simulink model "Three-phase Asynchronous Motor_Speed Regulation"  (R2017b)
settings: Solver=ode23tb  StartTime=0.0  StopTime=9  MaxStep=1e-4  RelTol=1e-3
libraries: powerlib x51, powerlib_meascontrol x1, simulink x1
settings Model: Creator=13248  LastModifiedBy=13248
settings DebuggingCC: UnconnectedInputMsg=none  UnconnectedOutputMsg=none  UnconnectedLineMsg=none

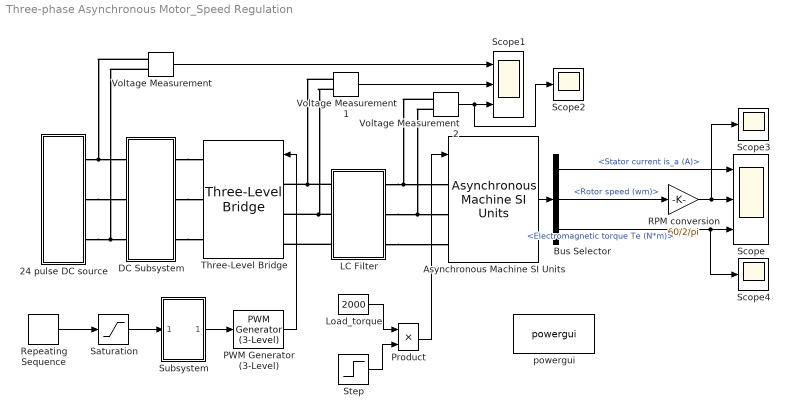
== system Three-phase Asynchronous Motor_Speed Regulation ==
  " DC Subsystem" : Subsystem
  24 pulse DC source : Subsystem
  Asynchronous Machine SI Units : powerlib/Machines/Asynchronous Machine SI Units  RotorType=Squirrel-cage  PresetModel=No  MechanicalLoad=Torque Tm  ShowDetailedParameters=on  ReferenceFrame=Rotor  Units=SI  MeasurementBus=off  NominalParameters=[500e3 6000 50]  Stator=[2 7/314]  Rotor=[1.9 5/314]  Cage1=[0.4155 0.002066]  Cage2=[0.4168 0.0003495]  Lm=235/314  Mechanical=[48 0 2]  PolePairs=2  InitialConditions=[1,0 0,0,0 0,0,0]  SimulateSaturation=off  Saturation=[14.03593122, 27.81365428, 53.79336849, 72.68890987, 97.98006896, 148.6815601, 215.7428561, 302.9841135, 428.7778367 ; 230, 322, 414, 460, 506, 552, 598, 644, 690]  LoadFlowParameters=1492000  TsPowergui=0  TsBlock=-1  IterativeModel=Trapezoidal non iterative  IterativeDiscreteModel=Trapezoidal non iterative  Pmec=1.492e+006
  Bus Selector : BusSelector  OutputSignals=Stator measurements.Stator current is_a (A),Mechanical.Rotor speed (wm),Mechanical.Electromagnetic torque Te (N*m)
  LC Filter : Subsystem
  Load_torque : Constant  Value=2000
  PWM Generator (3-Level) : powerlib_meascontrol/Pulse & Signal Generators/PWM Generator (3-Level)  ModulatorType=Three-phase bridge (12 pulses)  ModulatorMode=Unsynchronized  nF=27  Fc=18*50  ModulatingSignals=off  m=0.8  Freq=60  Phase=0  Ts=0
      settings: SourceProductName=Simscape Power Systems  SourceProductBaseCode=PS
  Product : Product
  RPM conversion : Gain  Gain=60/2/pi
  Repeating Sequence : simulink/Sources/Repeating Sequence  rep_seq_t=[0,0.5,2.5,2.51,5,5.01,10]  rep_seq_y=[0 15 15 35 35 50 50]
  Saturation : Saturate  UpperLimit=60  LowerLimit=0
  Scope : Scope  NumInputPorts=3
  Scope1 : Scope  NumInputPorts=3
  Scope2 : Scope
  Scope3 : Scope
  Scope4 : Scope
  Step : Step  Time=1.5  SampleTime=0
  Subsystem : Subsystem
  Three-Level Bridge : powerlib/Power Electronics/Three-Level Bridge  Arms=3  SnubberResistance=1e6  SbubberCapacitance=inf  Device=GTO / Diodes  Ron=1e-4  ForwardVoltages="[  1  1  ]"  Measurements=None
      settings: SourceProductName=Simscape Power Systems  SourceProductBaseCode=PS
  Voltage Measurement : powerlib/Measurements/Voltage Measurement  PhasorSimulation=off  OutputType=Complex  PSBequivalent=0
  Voltage Measurement1 : powerlib/Measurements/Voltage Measurement  PhasorSimulation=off  OutputType=Complex  PSBequivalent=0
  Voltage Measurement2 : powerlib/Measurements/Voltage Measurement  PhasorSimulation=off  OutputType=Complex  PSBequivalent=0
  powergui : powerlib/powergui  Priority=1  SimulationMode=Discrete  SampleTime=5.144e-6  frequency=60  Iterations=50  frequencyindice=50  Pbase=100e6  ErrMax=1e-4  UnitsV=kV  UnitsW=MW  buscounter=0  FunctionMessages=off  echomessages=off  EnableUseOfTLC=off  CurrentSourceSwitches=off  DisableSnubberDevices=off  DisableRonSwitches=off  DisableVfSwitches=off  DisplayEquations=off  SolverType=Tustin/Backward Euler (TBE)  Interpol=off  ExternalGateDelay=off  methode=off  Ts=100  x0status=steady  SPID=on  SwTol=0  HookPort=off  RestoreLinks=warning  ResistiveCurrentMeasurement=off  Frange=[0:2:500]  Ylog=off  Xlog=on  ShowGrid=off  save=off  variable=ZData  structure=0  ZoomFFT=off  StartTime=0.0  cycles=1  DisplayStyle=1  fundamental=60  FreqAxis=off  MaxFrequency=1000  frequencyindicesteady=1  RmsSteady=1  display=off
  wires:
  Bus Selector/2 -> RPM conversion/1  "<Rotor speed (wm)>"
  RPM conversion/1 -> Scope3/1, Scope/2
  Bus Selector/3 -> Scope/3, Scope4/1  "<Electromagnetic torque Te (N*m)>"
  Bus Selector/1 -> Scope/1  "<Stator current is_a (A)>"
  Repeating Sequence/1 -> Saturation/1
  Saturation/1 -> Subsystem/1(Cmd)
  Subsystem/1(Ust) -> PWM Generator (3-Level)/1
  PWM Generator (3-Level)/1 -> Three-Level Bridge/1
  Asynchronous Machine SI Units/1 -> Bus Selector/1
  Product/1 -> Asynchronous Machine SI Units/1
  Load_torque/1 -> Product/1
  Step/1 -> Product/2
  Voltage Measurement/1 -> Scope1/1
  Voltage Measurement1/1 -> Scope1/2
  Voltage Measurement2/1 -> Scope2/1, Scope1/3
  connections:
  24 pulse DC source/RConn1 -- Voltage Measurement/LConn1 -- " DC Subsystem"/LConn1
  24 pulse DC source/RConn2 -- " DC Subsystem"/LConn2
  24 pulse DC source/RConn3 -- Voltage Measurement/LConn2 -- " DC Subsystem"/LConn3
  " DC Subsystem"/RConn1 -- Three-Level Bridge/RConn1
  " DC Subsystem"/RConn2 -- Three-Level Bridge/RConn2
  " DC Subsystem"/RConn3 -- Three-Level Bridge/RConn3
  LC Filter/LConn1 -- Three-Level Bridge/LConn1 -- Voltage Measurement1/LConn1
  LC Filter/LConn2 -- Three-Level Bridge/LConn2 -- Voltage Measurement1/LConn2
  LC Filter/LConn3 -- Three-Level Bridge/LConn3
  LC Filter/RConn1 -- Voltage Measurement2/LConn1 -- Asynchronous Machine SI Units/LConn1
  LC Filter/RConn2 -- Voltage Measurement2/LConn2 -- Asynchronous Machine SI Units/LConn2
  LC Filter/RConn3 -- Asynchronous Machine SI Units/LConn3

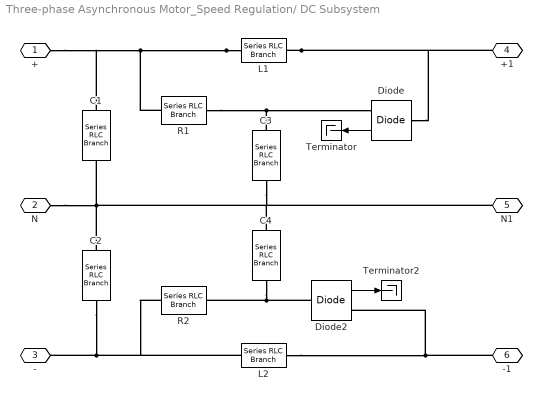
== system Three-phase Asynchronous Motor_Speed Regulation/ DC Subsystem ==
  C1 : powerlib/Elements/Series RLC Branch  LConnTagsString=__new0  RConnTagsString=__new0  BranchType=C  Resistance=0.5  Inductance=15e-6  SetiL0=off  InitialCurrent=0  Capacitance=960e-6  Setx0=off  InitialVoltage=0  Measurements=None
  C2 : powerlib/Elements/Series RLC Branch  LConnTagsString=__new0  RConnTagsString=__new0  BranchType=C  Resistance=0.5  Inductance=15e-6  SetiL0=off  InitialCurrent=0  Capacitance=960e-6  Setx0=off  InitialVoltage=0  Measurements=None
  C3 : powerlib/Elements/Series RLC Branch  LConnTagsString=__new0  RConnTagsString=__new0  BranchType=C  Resistance=0.5  Inductance=15e-6  SetiL0=off  InitialCurrent=0  Capacitance=10e-6  Setx0=off  InitialVoltage=0  Measurements=None
  C4 : powerlib/Elements/Series RLC Branch  LConnTagsString=__new0  RConnTagsString=__new0  BranchType=C  Resistance=0.5  Inductance=15e-6  SetiL0=off  InitialCurrent=0  Capacitance=10e-6  Setx0=off  InitialVoltage=0  Measurements=None
  Diode : powerlib/Power Electronics/Diode  Ron=0.001  Lon=0  Vf=0.8  IC=0  UseSnubber=0  Rs=500  Cs=250e-9  Measurements=on
  Diode2 : powerlib/Power Electronics/Diode  Ron=0.001  Lon=0  Vf=0.8  IC=0  UseSnubber=0  Rs=500  Cs=250e-9  Measurements=on
  L1 : powerlib/Elements/Series RLC Branch  LConnTagsString=__new0  RConnTagsString=__new0  BranchType=L  Resistance=1  Inductance=15e-6  SetiL0=off  InitialCurrent=0  Capacitance=1e-6  Setx0=off  InitialVoltage=0  Measurements=None
  L2 : powerlib/Elements/Series RLC Branch  LConnTagsString=__new0  RConnTagsString=__new0  BranchType=L  Resistance=1  Inductance=15e-6  SetiL0=off  InitialCurrent=0  Capacitance=1e-6  Setx0=off  InitialVoltage=0  Measurements=None
  R1 : powerlib/Elements/Series RLC Branch  LConnTagsString=__new0  RConnTagsString=__new0  BranchType=R  Resistance=0.5  Inductance=15e-6  SetiL0=off  InitialCurrent=0  Capacitance=1e-6  Setx0=off  InitialVoltage=0  Measurements=None
  R2 : powerlib/Elements/Series RLC Branch  LConnTagsString=__new0  RConnTagsString=__new0  BranchType=R  Resistance=0.5  Inductance=15e-6  SetiL0=off  InitialCurrent=0  Capacitance=1e-6  Setx0=off  InitialVoltage=0  Measurements=None
  Terminator : Terminator
  Terminator2 : Terminator
  + : PMIOPort  Port=1  Side=Left
  N : PMIOPort  Port=2  Side=Left
  - : PMIOPort  Port=3  Side=Left
  +1 : PMIOPort  Port=4  Side=Right
  N1 : PMIOPort  Port=5  Side=Right
  -1 : PMIOPort  Port=6  Side=Right
  wires:
  Diode2/1 -> Terminator2/1
  Diode/1 -> Terminator/1
  connections:
  L1/RConn1 -- +1/RConn1 -- Diode/LConn1
  R1/RConn1 -- C3/LConn1 -- Diode/RConn1
  L1/LConn1 -- +/RConn1 -- C1/LConn1 -- R1/LConn1
  C2/RConn1 -- -/RConn1 -- R2/LConn1 -- L2/LConn1
  C4/RConn1 -- Diode2/LConn1 -- R2/RConn1
  C2/LConn1 -- N/RConn1 -- N1/RConn1 -- C4/LConn1 -- C3/RConn1 -- C1/RConn1
  L2/RConn1 -- -1/RConn1 -- Diode2/RConn1

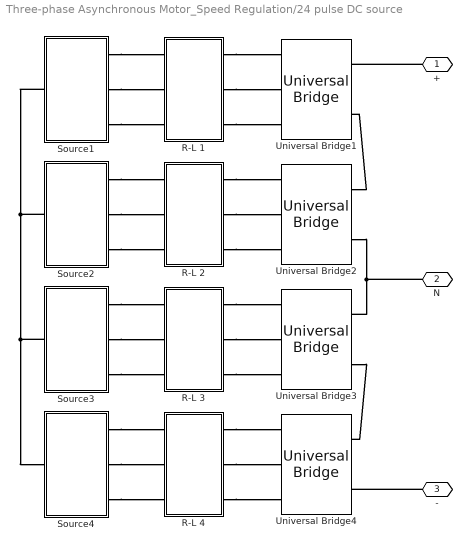
== system Three-phase Asynchronous Motor_Speed Regulation/24 pulse DC source ==
  R-L 1 : Subsystem
  R-L 2 : Subsystem
  R-L 3 : Subsystem
  R-L 4 : Subsystem
  Source1 : Subsystem
  Source2 : Subsystem
  Source3 : Subsystem
  Source4 : Subsystem
  Universal Bridge{1..4} (4 alike) : powerlib/Power Electronics/Universal Bridge  Arms=3  SnubberResistance=250  SnubberCapacitance=0.1e-6  Device=Diodes  Ron=0.01  Lon=0  ForwardVoltages="[  0  0  ]"  ForwardVoltage=0.8  GTOparameters=[ 10e-6 , 20e-6 ]  IGBTparameters=[ 1e-6 , 2e-6 ]  Measurements=Device currents  Measurements_2=None  converterType=Rectifier
  + : PMIOPort  Port=1  Side=Right
  N : PMIOPort  Port=2  Side=Right
  - : PMIOPort  Port=3  Side=Right
  connections:
  Source1/RConn2 -- R-L 1/LConn2
  R-L 2/RConn3 -- Universal Bridge2/LConn3
  R-L 2/RConn1 -- Universal Bridge2/LConn1
  Source1/LConn1 -- Source2/LConn1 -- Source3/LConn1 -- Source4/LConn1
  Universal Bridge3/RConn2 -- Universal Bridge4/RConn1
  Source1/RConn3 -- R-L 1/LConn3
  R-L 1/RConn3 -- Universal Bridge1/LConn3
  R-L 1/RConn2 -- Universal Bridge1/LConn2
  R-L 2/RConn2 -- Universal Bridge2/LConn2
  -/RConn1 -- Universal Bridge4/RConn2
  R-L 3/RConn1 -- Universal Bridge3/LConn1
  R-L 3/RConn2 -- Universal Bridge3/LConn2
  R-L 4/RConn1 -- Universal Bridge4/LConn1
  R-L 4/RConn2 -- Universal Bridge4/LConn2
  Universal Bridge2/RConn2 -- N/RConn1 -- Universal Bridge3/RConn1
  R-L 4/RConn3 -- Universal Bridge4/LConn3
  Source2/RConn2 -- R-L 2/LConn2
  Source4/RConn3 -- R-L 4/LConn3
  Source2/RConn1 -- R-L 2/LConn1
  R-L 1/RConn1 -- Universal Bridge1/LConn1
  Source4/RConn2 -- R-L 4/LConn2
  Source1/RConn1 -- R-L 1/LConn1
  R-L 3/RConn3 -- Universal Bridge3/LConn3
  +/RConn1 -- Universal Bridge1/RConn1
  Universal Bridge2/RConn1 -- Universal Bridge1/RConn2
  Source3/RConn3 -- R-L 3/LConn3
  Source4/RConn1 -- R-L 4/LConn1
  Source3/RConn2 -- R-L 3/LConn2
  Source3/RConn1 -- R-L 3/LConn1
  Source2/RConn3 -- R-L 2/LConn3

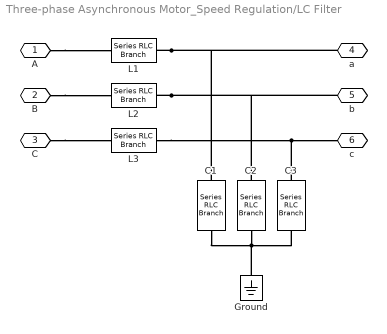
== system Three-phase Asynchronous Motor_Speed Regulation/LC Filter ==
  C1 : powerlib/Elements/Series RLC Branch  LConnTagsString=__new0  RConnTagsString=__new0  BranchType=C  Resistance=0.5  Inductance=15e-6  SetiL0=off  InitialCurrent=0  Capacitance=120e-6  Setx0=off  InitialVoltage=0  Measurements=None
  C2 : powerlib/Elements/Series RLC Branch  LConnTagsString=__new0  RConnTagsString=__new0  BranchType=C  Resistance=0.5  Inductance=15e-6  SetiL0=off  InitialCurrent=0  Capacitance=120e-6  Setx0=off  InitialVoltage=0  Measurements=None
  C3 : powerlib/Elements/Series RLC Branch  LConnTagsString=__new0  RConnTagsString=__new0  BranchType=C  Resistance=0.5  Inductance=15e-6  SetiL0=off  InitialCurrent=0  Capacitance=120e-6  Setx0=off  InitialVoltage=0  Measurements=None
  Ground : powerlib/Elements/Ground  LConnTagsString=a
  L1 : powerlib/Elements/Series RLC Branch  LConnTagsString=__new0  RConnTagsString=__new0  BranchType=L  Resistance=1  Inductance=0.002  SetiL0=off  InitialCurrent=0  Capacitance=1e-6  Setx0=off  InitialVoltage=0  Measurements=None
  L2 : powerlib/Elements/Series RLC Branch  LConnTagsString=__new0  RConnTagsString=__new0  BranchType=L  Resistance=1  Inductance=0.002  SetiL0=off  InitialCurrent=0  Capacitance=1e-6  Setx0=off  InitialVoltage=0  Measurements=None
  L3 : powerlib/Elements/Series RLC Branch  LConnTagsString=__new0  RConnTagsString=__new0  BranchType=L  Resistance=1  Inductance=0.002  SetiL0=off  InitialCurrent=0  Capacitance=1e-6  Setx0=off  InitialVoltage=0  Measurements=None
  A : PMIOPort  Port=1  Side=Left
  B : PMIOPort  Port=2  Side=Left
  C : PMIOPort  Port=3  Side=Left
  a : PMIOPort  Port=4  Side=Right
  b : PMIOPort  Port=5  Side=Right
  c : PMIOPort  Port=6  Side=Right
  connections:
  L3/RConn1 -- c/RConn1 -- C3/LConn1
  L1/RConn1 -- a/RConn1 -- C1/LConn1
  C2/RConn1 -- Ground/LConn1 -- C3/RConn1 -- C1/RConn1
  L2/RConn1 -- b/RConn1 -- C2/LConn1
  B/RConn1 -- L2/LConn1
  A/RConn1 -- L1/LConn1
  C/RConn1 -- L3/LConn1

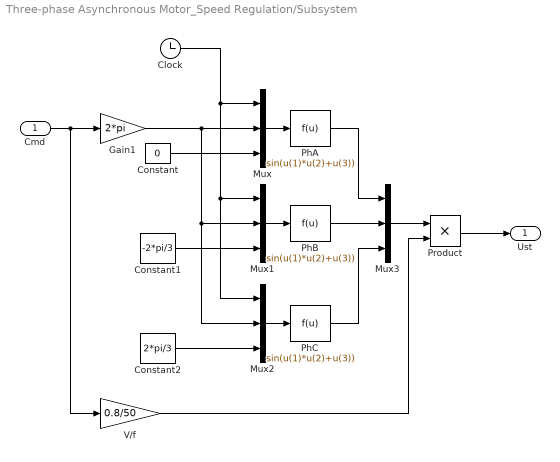
== system Three-phase Asynchronous Motor_Speed Regulation/Subsystem ==
  Cmd : Inport
  Clock : Clock
  Constant : Constant  Value=0
  Constant1 : Constant  Value=-2*pi/3
  Constant2 : Constant  Value=2*pi/3
  Gain1 : Gain  Gain=2*pi
  Mux{,1..3} (4 alike) : Mux  Inputs=3
  PhA : Fcn  Expr=sin(u(1)*u(2)+u(3))
  PhB : Fcn  Expr=sin(u(1)*u(2)+u(3))
  PhC : Fcn  Expr=sin(u(1)*u(2)+u(3))
  Product : Product
  V/f : Gain  Gain=0.8/50
  Ust : Outport
  wires:
  V/f/1 -> Product/2
  Constant2/1 -> Mux2/3
  Product/1 -> Ust/1
  Constant/1 -> Mux/3
  Clock/1 -> Mux2/1, Mux1/1, Mux/1
  PhC/1 -> Mux3/3
  Cmd/1 -> V/f/1, Gain1/1
  Mux3/1 -> Product/1
  Mux1/1 -> PhB/1
  Constant1/1 -> Mux1/3
  Mux2/1 -> PhC/1
  PhB/1 -> Mux3/2
  PhA/1 -> Mux3/1
  Mux/1 -> PhA/1
  Gain1/1 -> Mux2/2, Mux1/2, Mux/2

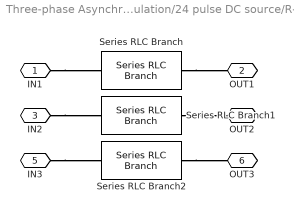
== system Three-phase Asynchronous Motor_Speed Regulation/24 pulse DC source/R-L 1 ==
  Series RLC Branch : powerlib/Elements/Series RLC Branch  LConnTagsString=__new0  RConnTagsString=__new0  BranchType=RL  Resistance=0.9  Inductance=0.002  SetiL0=off  InitialCurrent=0  Capacitance=1e-6  Setx0=off  InitialVoltage=0  Measurements=None
  Series RLC Branch1 : powerlib/Elements/Series RLC Branch  LConnTagsString=__new0  RConnTagsString=__new0  BranchType=RL  Resistance=0.9  Inductance=0.002  SetiL0=off  InitialCurrent=0  Capacitance=1e-6  Setx0=off  InitialVoltage=0  Measurements=None
  Series RLC Branch2 : powerlib/Elements/Series RLC Branch  LConnTagsString=__new0  RConnTagsString=__new0  BranchType=RL  Resistance=0.9  Inductance=0.002  SetiL0=off  InitialCurrent=0  Capacitance=1e-6  Setx0=off  InitialVoltage=0  Measurements=None
  IN1 : PMIOPort  Port=1  Side=Left
  OUT1 : PMIOPort  Port=2  Side=Right
  IN2 : PMIOPort  Port=3  Side=Left
  OUT2 : PMIOPort  Port=4  Side=Right
  IN3 : PMIOPort  Port=5  Side=Left
  OUT3 : PMIOPort  Port=6  Side=Right
  connections:
  IN2/RConn1 -- Series RLC Branch1/LConn1
  Series RLC Branch1/RConn1 -- OUT2/RConn1
  IN1/RConn1 -- Series RLC Branch/LConn1
  Series RLC Branch/RConn1 -- OUT1/RConn1
  IN3/RConn1 -- Series RLC Branch2/LConn1
  Series RLC Branch2/RConn1 -- OUT3/RConn1

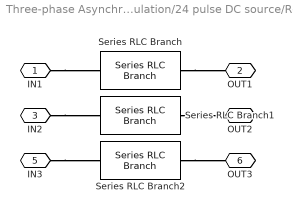
== system Three-phase Asynchronous Motor_Speed Regulation/24 pulse DC source/R-L 2 ==
  Series RLC Branch : powerlib/Elements/Series RLC Branch  LConnTagsString=__new0  RConnTagsString=__new0  BranchType=RL  Resistance=0.9  Inductance=0.002  SetiL0=off  InitialCurrent=0  Capacitance=1e-6  Setx0=off  InitialVoltage=0  Measurements=None
  Series RLC Branch1 : powerlib/Elements/Series RLC Branch  LConnTagsString=__new0  RConnTagsString=__new0  BranchType=RL  Resistance=0.9  Inductance=0.002  SetiL0=off  InitialCurrent=0  Capacitance=1e-6  Setx0=off  InitialVoltage=0  Measurements=None
  Series RLC Branch2 : powerlib/Elements/Series RLC Branch  LConnTagsString=__new0  RConnTagsString=__new0  BranchType=RL  Resistance=0.9  Inductance=0.002  SetiL0=off  InitialCurrent=0  Capacitance=1e-6  Setx0=off  InitialVoltage=0  Measurements=None
  IN1 : PMIOPort  Port=1  Side=Left
  OUT1 : PMIOPort  Port=2  Side=Right
  IN2 : PMIOPort  Port=3  Side=Left
  OUT2 : PMIOPort  Port=4  Side=Right
  IN3 : PMIOPort  Port=5  Side=Left
  OUT3 : PMIOPort  Port=6  Side=Right
  connections:
  IN2/RConn1 -- Series RLC Branch1/LConn1
  Series RLC Branch1/RConn1 -- OUT2/RConn1
  IN1/RConn1 -- Series RLC Branch/LConn1
  Series RLC Branch/RConn1 -- OUT1/RConn1
  IN3/RConn1 -- Series RLC Branch2/LConn1
  Series RLC Branch2/RConn1 -- OUT3/RConn1

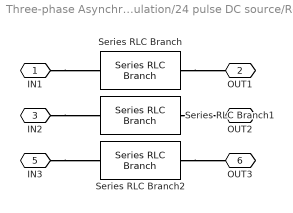
== system Three-phase Asynchronous Motor_Speed Regulation/24 pulse DC source/R-L 3 ==
  Series RLC Branch : powerlib/Elements/Series RLC Branch  LConnTagsString=__new0  RConnTagsString=__new0  BranchType=RL  Resistance=0.9  Inductance=0.002  SetiL0=off  InitialCurrent=0  Capacitance=1e-6  Setx0=off  InitialVoltage=0  Measurements=None
  Series RLC Branch1 : powerlib/Elements/Series RLC Branch  LConnTagsString=__new0  RConnTagsString=__new0  BranchType=RL  Resistance=0.9  Inductance=0.002  SetiL0=off  InitialCurrent=0  Capacitance=1e-6  Setx0=off  InitialVoltage=0  Measurements=None
  Series RLC Branch2 : powerlib/Elements/Series RLC Branch  LConnTagsString=__new0  RConnTagsString=__new0  BranchType=RL  Resistance=0.9  Inductance=0.002  SetiL0=off  InitialCurrent=0  Capacitance=1e-6  Setx0=off  InitialVoltage=0  Measurements=None
  IN1 : PMIOPort  Port=1  Side=Left
  OUT1 : PMIOPort  Port=2  Side=Right
  IN2 : PMIOPort  Port=3  Side=Left
  OUT2 : PMIOPort  Port=4  Side=Right
  IN3 : PMIOPort  Port=5  Side=Left
  OUT3 : PMIOPort  Port=6  Side=Right
  connections:
  IN2/RConn1 -- Series RLC Branch1/LConn1
  Series RLC Branch1/RConn1 -- OUT2/RConn1
  IN1/RConn1 -- Series RLC Branch/LConn1
  Series RLC Branch/RConn1 -- OUT1/RConn1
  IN3/RConn1 -- Series RLC Branch2/LConn1
  Series RLC Branch2/RConn1 -- OUT3/RConn1

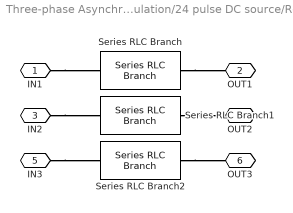
== system Three-phase Asynchronous Motor_Speed Regulation/24 pulse DC source/R-L 4 ==
  Series RLC Branch : powerlib/Elements/Series RLC Branch  LConnTagsString=__new0  RConnTagsString=__new0  BranchType=RL  Resistance=0.9  Inductance=0.002  SetiL0=off  InitialCurrent=0  Capacitance=1e-6  Setx0=off  InitialVoltage=0  Measurements=None
  Series RLC Branch1 : powerlib/Elements/Series RLC Branch  LConnTagsString=__new0  RConnTagsString=__new0  BranchType=RL  Resistance=0.9  Inductance=0.002  SetiL0=off  InitialCurrent=0  Capacitance=1e-6  Setx0=off  InitialVoltage=0  Measurements=None
  Series RLC Branch2 : powerlib/Elements/Series RLC Branch  LConnTagsString=__new0  RConnTagsString=__new0  BranchType=RL  Resistance=0.9  Inductance=0.002  SetiL0=off  InitialCurrent=0  Capacitance=1e-6  Setx0=off  InitialVoltage=0  Measurements=None
  IN1 : PMIOPort  Port=1  Side=Left
  OUT1 : PMIOPort  Port=2  Side=Right
  IN2 : PMIOPort  Port=3  Side=Left
  OUT2 : PMIOPort  Port=4  Side=Right
  IN3 : PMIOPort  Port=5  Side=Left
  OUT3 : PMIOPort  Port=6  Side=Right
  connections:
  IN2/RConn1 -- Series RLC Branch1/LConn1
  Series RLC Branch1/RConn1 -- OUT2/RConn1
  IN1/RConn1 -- Series RLC Branch/LConn1
  Series RLC Branch/RConn1 -- OUT1/RConn1
  IN3/RConn1 -- Series RLC Branch2/LConn1
  Series RLC Branch2/RConn1 -- OUT3/RConn1

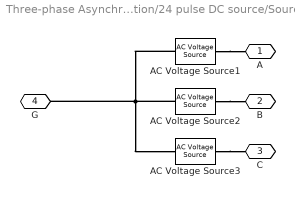
== system Three-phase Asynchronous Motor_Speed Regulation/24 pulse DC source/Source1 ==
  AC Voltage Source1 : powerlib/Electrical Sources/AC Voltage Source  Amplitude=6600/sqrt(3)*sqrt(2)  Phase=0  Frequency=50  SampleTime=0  Measurements=None  BusType=swing  Pref=10e3  Qref=0  Qmin=-inf  Qmax=+inf
  AC Voltage Source2 : powerlib/Electrical Sources/AC Voltage Source  Amplitude=6600/sqrt(3)*sqrt(2)  Phase=-120  Frequency=50  SampleTime=0  Measurements=None  BusType=swing  Pref=10e3  Qref=0  Qmin=-inf  Qmax=+inf
  AC Voltage Source3 : powerlib/Electrical Sources/AC Voltage Source  Amplitude=6600/sqrt(3)*sqrt(2)  Phase=120  Frequency=50  SampleTime=0  Measurements=None  BusType=swing  Pref=10e3  Qref=0  Qmin=-inf  Qmax=+inf
  A : PMIOPort  Port=1  Side=Right
  B : PMIOPort  Port=2  Side=Right
  C : PMIOPort  Port=3  Side=Right
  G : PMIOPort  Port=4  Side=Left
  connections:
  AC Voltage Source1/LConn1 -- G/RConn1 -- AC Voltage Source2/LConn1 -- AC Voltage Source3/LConn1
  AC Voltage Source3/RConn1 -- C/RConn1
  AC Voltage Source2/RConn1 -- B/RConn1
  AC Voltage Source1/RConn1 -- A/RConn1

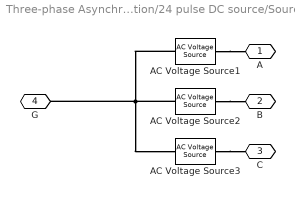
== system Three-phase Asynchronous Motor_Speed Regulation/24 pulse DC source/Source2 ==
  AC Voltage Source1 : powerlib/Electrical Sources/AC Voltage Source  Amplitude=6600/sqrt(3)*sqrt(2)  Phase=15  Frequency=50  SampleTime=0  Measurements=None  BusType=swing  Pref=10e3  Qref=0  Qmin=-inf  Qmax=+inf
  AC Voltage Source2 : powerlib/Electrical Sources/AC Voltage Source  Amplitude=6600/sqrt(3)*sqrt(2)  Phase=-105  Frequency=50  SampleTime=0  Measurements=None  BusType=swing  Pref=10e3  Qref=0  Qmin=-inf  Qmax=+inf
  AC Voltage Source3 : powerlib/Electrical Sources/AC Voltage Source  Amplitude=6600/sqrt(3)*sqrt(2)  Phase=135  Frequency=50  SampleTime=0  Measurements=None  BusType=swing  Pref=10e3  Qref=0  Qmin=-inf  Qmax=+inf
  A : PMIOPort  Port=1  Side=Right
  B : PMIOPort  Port=2  Side=Right
  C : PMIOPort  Port=3  Side=Right
  G : PMIOPort  Port=4  Side=Left
  connections:
  AC Voltage Source1/LConn1 -- G/RConn1 -- AC Voltage Source2/LConn1 -- AC Voltage Source3/LConn1
  AC Voltage Source3/RConn1 -- C/RConn1
  AC Voltage Source2/RConn1 -- B/RConn1
  AC Voltage Source1/RConn1 -- A/RConn1

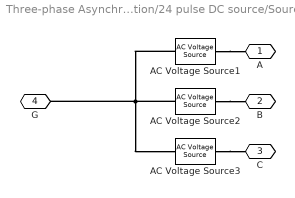
== system Three-phase Asynchronous Motor_Speed Regulation/24 pulse DC source/Source3 ==
  AC Voltage Source1 : powerlib/Electrical Sources/AC Voltage Source  Amplitude=6600/sqrt(3)*sqrt(2)  Phase=30  Frequency=50  SampleTime=0  Measurements=None  BusType=swing  Pref=10e3  Qref=0  Qmin=-inf  Qmax=+inf
  AC Voltage Source2 : powerlib/Electrical Sources/AC Voltage Source  Amplitude=6600/sqrt(3)*sqrt(2)  Phase=-90  Frequency=50  SampleTime=0  Measurements=None  BusType=swing  Pref=10e3  Qref=0  Qmin=-inf  Qmax=+inf
  AC Voltage Source3 : powerlib/Electrical Sources/AC Voltage Source  Amplitude=6600/sqrt(3)*sqrt(2)  Phase=150  Frequency=50  SampleTime=0  Measurements=None  BusType=swing  Pref=10e3  Qref=0  Qmin=-inf  Qmax=+inf
  A : PMIOPort  Port=1  Side=Right
  B : PMIOPort  Port=2  Side=Right
  C : PMIOPort  Port=3  Side=Right
  G : PMIOPort  Port=4  Side=Left
  connections:
  AC Voltage Source1/LConn1 -- G/RConn1 -- AC Voltage Source2/LConn1 -- AC Voltage Source3/LConn1
  AC Voltage Source3/RConn1 -- C/RConn1
  AC Voltage Source2/RConn1 -- B/RConn1
  AC Voltage Source1/RConn1 -- A/RConn1

== system Three-phase Asynchronous Motor_Speed Regulation/24 pulse DC source/Source4 ==
  AC Voltage Source1 : powerlib/Electrical Sources/AC Voltage Source  Amplitude=6600/sqrt(3)*sqrt(2)  Phase=45  Frequency=50  SampleTime=0  Measurements=None  BusType=swing  Pref=10e3  Qref=0  Qmin=-inf  Qmax=+inf
  AC Voltage Source2 : powerlib/Electrical Sources/AC Voltage Source  Amplitude=6600/sqrt(3)*sqrt(2)  Phase=-75  Frequency=50  SampleTime=0  Measurements=None  BusType=swing  Pref=10e3  Qref=0  Qmin=-inf  Qmax=+inf
  AC Voltage Source3 : powerlib/Electrical Sources/AC Voltage Source  Amplitude=6600/sqrt(3)*sqrt(2)  Phase=165  Frequency=50  SampleTime=0  Measurements=None  BusType=swing  Pref=10e3  Qref=0  Qmin=-inf  Qmax=+inf
  A : PMIOPort  Port=1  Side=Right
  B : PMIOPort  Port=2  Side=Right
  C : PMIOPort  Port=3  Side=Right
  G : PMIOPort  Port=4  Side=Left
  connections:
  AC Voltage Source1/LConn1 -- G/RConn1 -- AC Voltage Source2/LConn1 -- AC Voltage Source3/LConn1
  AC Voltage Source3/RConn1 -- C/RConn1
  AC Voltage Source2/RConn1 -- B/RConn1
  AC Voltage Source1/RConn1 -- A/RConn1
